simulink model "x4_oqpsk"  (R2023b)
settings: Solver=VariableStepAuto  StartTime=0.0  StopTime=1000  RelTol=1e-3
libraries: commdigbbndpm3 x2, commrandsrc3 x1, commsink2 x1, commutil2 x1
settings Model: Creator=The MathWorks, Inc.  LastModifiedBy=Abhi Singh
settings SolverCC: AlgebraicLoopSolver=TrustRegion
settings DataIOCC: ReturnWorkspaceOutputs=off
settings DebuggingCC: UnconnectedInputMsg=warning  UnconnectedOutputMsg=warning  UnconnectedLineMsg=warning  ArithmeticOperatorsInVariantConditions=warning
settings ModelReferenceCC: EnableRefExpFcnMdlSchedulingChecks=on
settings SFSimCC: SimUseLocalCustomCode=off  CustomCodeUndefinedFunction=UseInterfaceOnly
settings RTWCC: RTWUseLocalCustomCode=off  DLArmComputeVersion=19.05

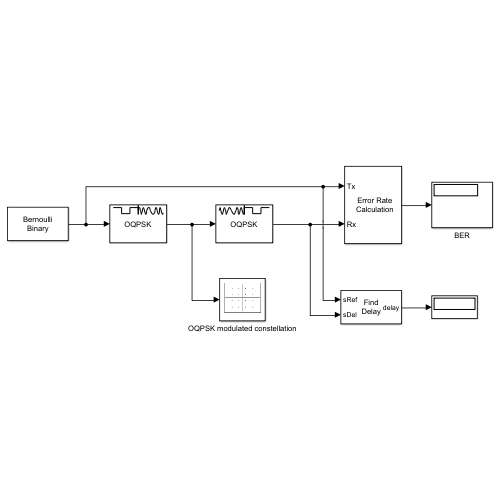
[thumbnail: Simulink's stored preview of the top-level diagram]
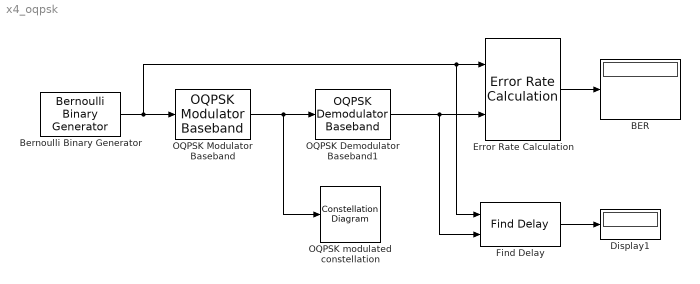
== system x4_oqpsk ==
  BER : Display
  Bernoulli Binary Generator : commrandsrc3/Bernoulli Binary Generator  ProbabilityOfZero=0.5  SeedSource=Auto  Seed=0  SampleTime=0.5e-3  SamplesPerFrame=1000  OutputDataType=double  SimulateUsing=Interpreted execution
  Display1 : Display
  Error Rate Calculation : commsink2/Error Rate Calculation  N=2  st_delay=0  cp_mode=Entire frame  subframe=[]  PMode=Port  WsName=ErrorVec  RsMode2=off  stop=off  numErr=100  maxBits=1e6
  Find Delay : commutil2/Find Delay  corrLength=200  chgSigOP=off  stopUpdate=off  numConstDelay=3
  OQPSK Demodulator Baseband1 : commdigbbndpm3/OQPSK Demodulator Baseband  OutType=Bit  Ph=0  Mapping=Gray  pulseShape=Half sine  num=[0.7071, 0.7071]  rolloff=0.2  filterSpan=10  sps=4  RateOptions=Enforce single-rate processing  outDtype2=double
  OQPSK Modulator Baseband : commdigbbndpm3/OQPSK Modulator Baseband  InType=Bit  Mapping=Gray  Ph=0  pulseShape=Half sine  num=[0.5, 0.5]  rolloff=0.2  filterSpan=10  sps=4  RateOptions=Enforce single-rate processing  outDtype=double
  OQPSK modulated constellation : ConstellationDiagram  WindowPosition=[58 1130 359 366]  SamplesPerSymbol=2  XLimits=[-1 1]  YLimits=[-1.25 1.25]  DefaultConfigurationName=comm.scopes.ConstellationDiagramBlockCfg
  wires:
  Bernoulli Binary Generator/1 -> Error Rate Calculation/1, Find Delay/1, OQPSK Modulator Baseband/1
  OQPSK Demodulator Baseband1/1 -> Error Rate Calculation/2, Find Delay/2
  Error Rate Calculation/1 -> BER/1
  Find Delay/1 -> Display1/1
  OQPSK Modulator Baseband/1 -> OQPSK Demodulator Baseband1/1, OQPSK modulated constellation/1
